simulink model "Robot"  (R2018a)
settings: Solver=VariableStepAuto  StartTime=0.0  StopTime=inf  FixedStep=1e-4  RelTol=1e-3  EnableMultiTasking=on
values from neighbouring files (symbols this model uses):
  CM730_acc_center = (4 * 9.80665)    (= 39.2266)    [CM730.m]
  CM730_acc_gain = 512 / CM730_acc_center    (= 13.0523675261)    [CM730.m]
  CM730_gyro_center = (1600 / 360 * 2 * pi)    (= 27.9252680319)    [CM730.m]
  CM730_gyro_gain = 512 / CM730_gyro_center    (= 18.3346494442)    [CM730.m]
  CM730_sample_time = 1e-3    (= 0.001)    [CM730.m]
  FSR_max = 254    [FSR.m]
  FSR_no_load = 255    [FSR.m]
  FSR_sample_time = 0.001    [FSR.m]
  FSR_scale = 1000    [FSR.m]
  g = 0    [Euler.m]
  MX106_Te = 1/1000    (= 0.001)    [MX106_init.m]
  MX28_inertia = 9e-8 * MX28_reduction^2    (= 0.0033385284)    [MX28_init.m]
  MX28_Te = 1/1000    (= 0.001)    [MX28_init.m]
  posZero_ID1 = posZero(1)    [Robot_init.m]
  posZero_ID10 = posZero(14)    [Robot_init.m]
  posZero_ID11 = posZero(9)    [Robot_init.m]
  posZero_ID12 = posZero(15)    [Robot_init.m]
  posZero_ID13 = posZero(10)    [Robot_init.m]
  posZero_ID14 = posZero(16)    [Robot_init.m]
  posZero_ID15 = posZero(11)    [Robot_init.m]
  posZero_ID16 = posZero(17)    [Robot_init.m]
  posZero_ID17 = posZero(12)    [Robot_init.m]
  posZero_ID18 = posZero(18)    [Robot_init.m]
  posZero_ID19 = posZero(19)    [Robot_init.m]
  posZero_ID2 = posZero(4)    [Robot_init.m]
  posZero_ID20 = posZero(20)    [Robot_init.m]
  posZero_ID3 = posZero(2)    [Robot_init.m]
  posZero_ID4 = posZero(5)    [Robot_init.m]
  posZero_ID5 = posZero(3)    [Robot_init.m]
  posZero_ID6 = posZero(6)    [Robot_init.m]
  posZero_ID7 = posZero(7)    [Robot_init.m]
  posZero_ID8 = posZero(13)    [Robot_init.m]
  posZero_ID9 = posZero(8)    [Robot_init.m]
  robot_chest_mass = 2385.0    (= 2385)    [Robot_init.m]
  robot_floor_friction_coeff = 0.6    [Robot_init.m]
  robot_floor_position_gain = -1e5    (= -100000)    [Robot_init.m]
  robot_floor_speed_gain = -1e3    (= -1000)    [Robot_init.m]
  robot_gravity = [0 0 0]    [Robot_init.m]
  robot_head_mass = 177.69    [Robot_init.m]
  robot_hip1_mass = 49.00    (= 49)    [Robot_init.m]
  robot_left_ankle_mass = 360.00    (= 360)    [Robot_init.m]
  robot_left_foot_mass = 267.00    (= 267)    [Robot_init.m]
  robot_left_forearm_mass = 248.00    (= 248)    [Robot_init.m]
  robot_left_hip2_mass = 358.00    (= 358)    [Robot_init.m]
  robot_left_lower_leg_mass = 129.00    (= 129)    [Robot_init.m]
  robot_left_shoulder_mass = 39.00    (= 39)    [Robot_init.m]
  robot_left_thigh_mass = 1263.00    (= 1263)    [Robot_init.m]
  robot_left_upper_arm_mass = 247.00    (= 247)    [Robot_init.m]
  robot_neck_mass = 90    [Robot_init.m]
  robot_right_ankle_mass = 360.00    (= 360)    [Robot_init.m]
  robot_right_foot_mass = 267.00    (= 267)    [Robot_init.m]
  robot_right_forearm_mass = 248.00    (= 248)    [Robot_init.m]
  robot_right_hip2_mass = 358.00    (= 358)    [Robot_init.m]
  robot_right_lower_leg_mass = 129.00    (= 129)    [Robot_init.m]
  robot_right_shoulder_mass = 39.00    (= 39)    [Robot_init.m]
  robot_right_thigh_mass = 263.00    (= 263)    [Robot_init.m]
  robot_right_upper_arm_mass = 247.00    (= 247)    [Robot_init.m]
  X = get(hObject,'Value')    [gui_kine.m]
  Y = get(hObject,'Value')    [gui_kine.m]
  Z = get(hObject,'Value')    [gui_kine.m]
libraries: sm_lib x167, fl_lib x128, nesl_utility x77, dspindex x1
(part 1 of 7)
settings Model: Creator=florent  LastModifiedBy=MRL
settings DataIOCC: SaveFormat=Array  SaveOutput=off  SignalLogging=off  DSMLogging=off  VisualizeSimOutput=off  SaveTime=off  OutputTimes=0:0.04:10
settings OptimizationCC: OptimizeBlockIOStorage=off  BufferReuse=off  GlobalBufferReuse=off  ExpressionFolding=off  LocalBlockOutputs=off  LifeSpan=inf  OptimizeDataStoreBuffers=off  BusAssignmentInplaceUpdate=off
settings DebuggingCC: SolverPrmCheckMsg=warning  StateNameClashWarn=warning  SFUnexpectedBacktrackingDiag=warning  SFNoUnconditionalDefaultTransitionDiag=warning  SFExecutionAtInitializationDiag=none
settings HardwareCC: ProdBitPerPointer=32  ProdBitPerSizeT=32  ProdBitPerPtrDiffT=32  ProdLargestAtomicFloat=None  ProdIntDivRoundTo=Undefined  ProdEndianess=Unspecified  ProdWordSize=32  ProdHWDeviceType=32-bit Generic
settings ModelReferenceCC: PropagateSignalLabelsOutOfModel=off
settings CodeAppCC: StateflowObjectComments=on
settings GRTTargetCC: TargetLangStandard=C89/C90 (ANSI)  GeneratePreprocessorConditionals=Disable all
settings ConfigComp: CovMetricSettings=dw  CovHtmlReporting=on  CovSaveCumulativeToWorkspaceVar=on  CovSaveSingleToWorkspaceVar=on  CovExternalEMLEnable=off  CovSFcnEnable=off
settings SimscapeCC: SimscapeNormalizeSystem=off
settings ConfigurationSet: Description=SimMechanics 2G
settings DiagnosticsConfigSet: SimMechanicsConflictingReferenceFrames=none

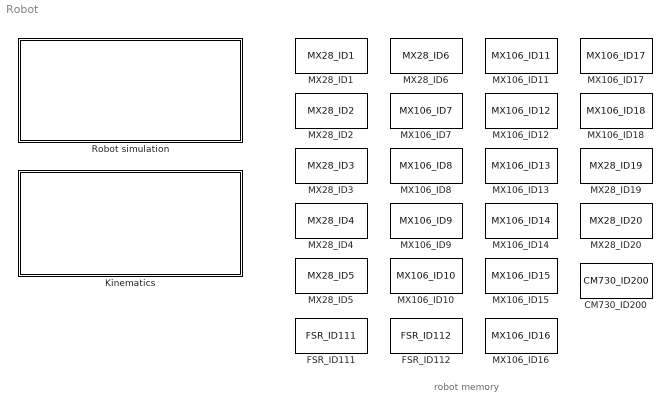
== system Robot ==
  note: robot memory
  CM730_ID200 : DataStoreMemory  DataStoreName=CM730_ID200  WriteAfterWriteMsg=error  InitialValue=CM730_default  VectorParams1D=off  ShowAdditionalParam=off  OutDataTypeStr=Bus: CM730_bus
  FSR_ID111 : DataStoreMemory  DataStoreName=FSR_ID111  WriteAfterWriteMsg=error  InitialValue=FSR_default  VectorParams1D=off  ShowAdditionalParam=off  OutDataTypeStr=Bus: FSR_bus
  FSR_ID112 : DataStoreMemory  DataStoreName=FSR_ID112  WriteAfterWriteMsg=error  InitialValue=FSR_default  VectorParams1D=off  ShowAdditionalParam=off  OutDataTypeStr=Bus: FSR_bus
  Kinematics : Subsystem
  MX106_ID10 : DataStoreMemory  DataStoreName=MX106_ID10  WriteAfterWriteMsg=error  InitialValue=MX106_default  VectorParams1D=off  ShowAdditionalParam=off  OutDataTypeStr=Bus: MX106_bus
  MX106_ID11 : DataStoreMemory  DataStoreName=MX106_ID11  WriteAfterWriteMsg=error  InitialValue=MX106_default  VectorParams1D=off  ShowAdditionalParam=off  OutDataTypeStr=Bus: MX106_bus
  MX106_ID12 : DataStoreMemory  DataStoreName=MX106_ID12  WriteAfterWriteMsg=error  InitialValue=MX106_default  VectorParams1D=off  ShowAdditionalParam=off  OutDataTypeStr=Bus: MX106_bus
  MX106_ID13 : DataStoreMemory  DataStoreName=MX106_ID13  WriteAfterWriteMsg=error  InitialValue=MX106_default  VectorParams1D=off  ShowAdditionalParam=off  OutDataTypeStr=Bus: MX106_bus
  MX106_ID14 : DataStoreMemory  DataStoreName=MX106_ID14  WriteAfterWriteMsg=error  InitialValue=MX106_default  VectorParams1D=off  ShowAdditionalParam=off  OutDataTypeStr=Bus: MX106_bus
  MX106_ID15 : DataStoreMemory  DataStoreName=MX106_ID15  WriteAfterWriteMsg=error  InitialValue=MX106_default  VectorParams1D=off  ShowAdditionalParam=off  OutDataTypeStr=Bus: MX106_bus
  MX106_ID16 : DataStoreMemory  DataStoreName=MX106_ID16  WriteAfterWriteMsg=error  InitialValue=MX106_default  VectorParams1D=off  ShowAdditionalParam=off  OutDataTypeStr=Bus: MX106_bus
  MX106_ID17 : DataStoreMemory  DataStoreName=MX106_ID17  WriteAfterWriteMsg=error  InitialValue=MX106_default  VectorParams1D=off  ShowAdditionalParam=off  OutDataTypeStr=Bus: MX106_bus
  MX106_ID18 : DataStoreMemory  DataStoreName=MX106_ID18  WriteAfterWriteMsg=error  InitialValue=MX106_default  VectorParams1D=off  ShowAdditionalParam=off  OutDataTypeStr=Bus: MX106_bus
  MX106_ID7 : DataStoreMemory  DataStoreName=MX106_ID7  WriteAfterWriteMsg=error  InitialValue=MX106_default  VectorParams1D=off  ShowAdditionalParam=off  OutDataTypeStr=Bus: MX106_bus
  MX106_ID8 : DataStoreMemory  DataStoreName=MX106_ID8  WriteAfterWriteMsg=error  InitialValue=MX106_default  VectorParams1D=off  ShowAdditionalParam=off  OutDataTypeStr=Bus: MX106_bus
  MX106_ID9 : DataStoreMemory  DataStoreName=MX106_ID9  WriteAfterWriteMsg=error  InitialValue=MX106_default  VectorParams1D=off  ShowAdditionalParam=off  OutDataTypeStr=Bus: MX106_bus
  MX28_ID1 : DataStoreMemory  DataStoreName=MX28_ID1  WriteAfterWriteMsg=error  InitialValue=MX28_default  VectorParams1D=off  ShowAdditionalParam=off  OutDataTypeStr=Bus: MX28_bus
  MX28_ID19 : DataStoreMemory  DataStoreName=MX28_ID19  WriteAfterWriteMsg=error  InitialValue=MX28_default  VectorParams1D=off  ShowAdditionalParam=off  OutDataTypeStr=Bus: MX28_bus
  MX28_ID2 : DataStoreMemory  DataStoreName=MX28_ID2  WriteAfterWriteMsg=error  InitialValue=MX28_default  VectorParams1D=off  ShowAdditionalParam=off  OutDataTypeStr=Bus: MX28_bus
  MX28_ID20 : DataStoreMemory  DataStoreName=MX28_ID20  WriteAfterWriteMsg=error  InitialValue=MX28_default  VectorParams1D=off  ShowAdditionalParam=off  OutDataTypeStr=Bus: MX28_bus
  MX28_ID3 : DataStoreMemory  DataStoreName=MX28_ID3  WriteAfterWriteMsg=error  InitialValue=MX28_default  VectorParams1D=off  ShowAdditionalParam=off  OutDataTypeStr=Bus: MX28_bus
  MX28_ID4 : DataStoreMemory  DataStoreName=MX28_ID4  WriteAfterWriteMsg=error  InitialValue=MX28_default  VectorParams1D=off  ShowAdditionalParam=off  OutDataTypeStr=Bus: MX28_bus
  MX28_ID5 : DataStoreMemory  DataStoreName=MX28_ID5  WriteAfterWriteMsg=error  InitialValue=MX28_default  VectorParams1D=off  ShowAdditionalParam=off  OutDataTypeStr=Bus: MX28_bus
  MX28_ID6 : DataStoreMemory  DataStoreName=MX28_ID6  WriteAfterWriteMsg=error  InitialValue=MX28_default  VectorParams1D=off  ShowAdditionalParam=off  OutDataTypeStr=Bus: MX28_bus
  Robot simulation : Subsystem

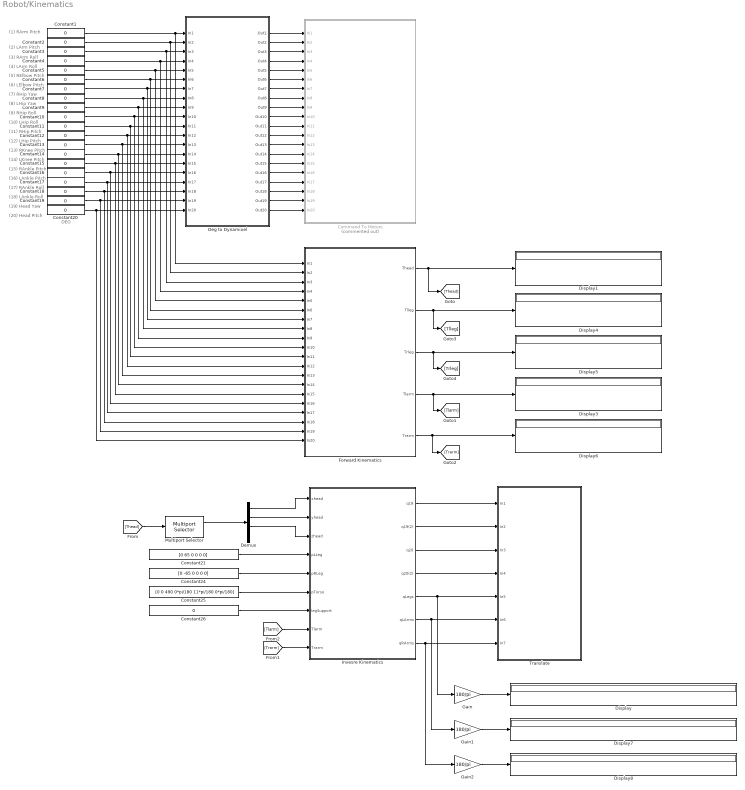
== system Robot/Kinematics ==
  note: (1) RArm Pitch
  note: (2) LArm Pitch
  note: (3) RArm Roll
  note: (4) LArm Roll
  note: (5) RElbow Pitch
  note: (6) LElbow Pitch
  note: (7) RHip Yaw
  note: (8) LHip Yaw
  note: (9) RHip Roll
  note: (10) LHip Roll
  note: (11) RHip Pitch
  note: (12) LHip Pitch
  note: (13) RKnee Pitch
  note: (14) LKnee Pitch
  note: (15) RAnkle Pitch
  note: (16) LAnkle Pitch
  note: (17) RAnkle Roll
  note: (18) LAnkle Roll
  note: (19) Head Yaw
  note: (20) Head Pitch
  note: DEG
  Command To Motors : Subsystem  Commented=on
  Constant{1..20} (20 alike) : Constant  Value=0  OutDataTypeStr=int16
  Constant21 : Constant  Value=[0 65 0 0 0 0]
  Constant24 : Constant  Value=[0 -65 0 0 0 0]
  Constant25 : Constant  Value="[0  0   490   0*pi/180   11*pi/180   0*pi/180]"
  Constant26 : Constant  Value=0
  Deg to Dynamixel : Subsystem
  Demux : Demux
  Display{,1,3..8} (8 alike) : Display
      Display1 settings: Format=bank
      Display3 settings: Format=bank
      Display4 settings: Format=bank
      Display5 settings: Format=bank
      Display6 settings: Format=bank
  Forward Kinematics : Subsystem
  Gain : Gain  Gain=180/pi
  Gain1 : Gain  Gain=180/pi
  Gain2 : Gain  Gain=180/pi
  Invesre Kinematics : Subsystem
  Multiport Selector : dspindex/Multiport Selector  rowsOrCols=Columns  idxCellArray={ 4,1}  idxErrMode=Clip Index
  Translate : Subsystem
  wires:
  Forward Kinematics/1(Thead) -> [Thead], Display1/1
  Forward Kinematics/2(Tlleg) -> Display4/1, [Tlleg]
  Forward Kinematics/3(Trleg) -> Display5/1, [Trleg]
  Constant1/1 -> Forward Kinematics/1(In1), Deg to Dynamixel/1(In1)
  Constant2/1 -> Forward Kinematics/2(In2), Deg to Dynamixel/2(In2)
  Constant3/1 -> Forward Kinematics/3(In3), Deg to Dynamixel/3(In3)
  Constant4/1 -> Forward Kinematics/4(In4), Deg to Dynamixel/4(In4)
  Constant5/1 -> Forward Kinematics/5(In5), Deg to Dynamixel/5(In5)
  Constant6/1 -> Forward Kinematics/6(In6), Deg to Dynamixel/6(In6)
  Constant7/1 -> Forward Kinematics/7(In7), Deg to Dynamixel/7(In7)
  Constant8/1 -> Forward Kinematics/8(In8), Deg to Dynamixel/8(In8)
  Constant9/1 -> Forward Kinematics/9(In9), Deg to Dynamixel/9(In9)
  Constant10/1 -> Forward Kinematics/10(In10), Deg to Dynamixel/10(In10)
  Constant11/1 -> Forward Kinematics/11(In11), Deg to Dynamixel/11(In11)
  Constant12/1 -> Forward Kinematics/12(In12), Deg to Dynamixel/12(In12)
  Constant13/1 -> Forward Kinematics/13(In13), Deg to Dynamixel/13(In13)
  Constant14/1 -> Forward Kinematics/14(In14), Deg to Dynamixel/14(In14)
  Constant15/1 -> Forward Kinematics/15(In15), Deg to Dynamixel/15(In15)
  Constant17/1 -> Forward Kinematics/17(In17), Deg to Dynamixel/17(In17)
  Constant18/1 -> Forward Kinematics/18(In18), Deg to Dynamixel/18(In18)
  Constant19/1 -> Forward Kinematics/19(In19), Deg to Dynamixel/19(In19)
  Deg to Dynamixel/1(Out1) -> Command To Motors/1(In1)
  Deg to Dynamixel/2(Out2) -> Command To Motors/2(In2)
  Deg to Dynamixel/3(Out3) -> Command To Motors/3(In3)
  Deg to Dynamixel/4(Out4) -> Command To Motors/4(In4)
  Deg to Dynamixel/5(Out5) -> Command To Motors/5(In5)
  Deg to Dynamixel/6(Out6) -> Command To Motors/6(In6)
  Deg to Dynamixel/7(Out7) -> Command To Motors/7(In7)
  Deg to Dynamixel/8(Out8) -> Command To Motors/8(In8)
  Deg to Dynamixel/9(Out9) -> Command To Motors/9(In9)
  Deg to Dynamixel/10(Out10) -> Command To Motors/10(In10)
  Deg to Dynamixel/11(Out11) -> Command To Motors/11(In11)
  Deg to Dynamixel/12(Out12) -> Command To Motors/12(In12)
  Deg to Dynamixel/13(Out13) -> Command To Motors/13(In13)
  Deg to Dynamixel/14(Out14) -> Command To Motors/14(In14)
  Deg to Dynamixel/15(Out15) -> Command To Motors/15(In15)
  Deg to Dynamixel/16(Out16) -> Command To Motors/16(In16)
  Deg to Dynamixel/17(Out17) -> Command To Motors/17(In17)
  Deg to Dynamixel/18(Out18) -> Command To Motors/18(In18)
  Deg to Dynamixel/19(Out19) -> Command To Motors/19(In19)
  Deg to Dynamixel/20(Out20) -> Command To Motors/20(In20)
  Constant16/1 -> Forward Kinematics/16(In16), Deg to Dynamixel/16(In16)
  [Thead] -> Multiport Selector/1
  Multiport Selector/1 -> Demux/1
  Demux/2 -> Invesre Kinematics/2(yhead)
  Demux/3 -> Invesre Kinematics/3(zhead)
  Invesre Kinematics/1(q19) -> Translate/1(In1)
  Invesre Kinematics/2(q19(2)) -> Translate/2(In2)
  Invesre Kinematics/3(q20) -> Translate/3(In3)
  Invesre Kinematics/4(q20(2)) -> Translate/4(In4)
  Demux/1 -> Invesre Kinematics/1(xhead)
  Constant20/1 -> Forward Kinematics/20(In20), Deg to Dynamixel/20(In20)
  Constant24/1 -> Invesre Kinematics/5(pRLeg)
  Constant25/1 -> Invesre Kinematics/6(pTorso)
  Constant26/1 -> Invesre Kinematics/7(legSupport)
  Invesre Kinematics/5(qLegs) -> Gain/1, Translate/5(In5)
  Gain/1 -> Display/1
  Constant21/1 -> Invesre Kinematics/4(pLLeg)
  Invesre Kinematics/6(qLArms) -> Gain1/1, Translate/6(In6)
  Invesre Kinematics/7(qRArms) -> Gain2/1, Translate/7(In7)
  Forward Kinematics/4(Tlarm) -> [Tlarm], Display3/1
  Forward Kinematics/5(Trarm) -> [Trarm], Display6/1
  Gain1/1 -> Display7/1
  Gain2/1 -> Display8/1
  [Trarm] -> Invesre Kinematics/9(Trarm)
  [Tlarm] -> Invesre Kinematics/8(Tlarm)

== system Robot/Robot simulation ==
  Chest : Subsystem
      mask init:
      | [ModelDir,~,~] = fileparts(which(gcs));
      | 
      | Block = [gcb '/Solid'];
      | STLFileName = [ModelDir filesep 'STL' filesep 'Chest.STL'];
      | if ~strcmp(get_param(Block,'ExtGeomFileName'),STLFileName)
      |     set_param(Block,'ExtGeomFileName',STLFileName);
      | end
  Free Fall Scope : Scope  Commented=on
  Free fall : sm_lib/Joints/6-DOF Joint  SenseConstraintForce=off  SenseConstraintForceX=off  SenseConstraintForceY=off  SenseConstraintForceZ=off  SenseConstraintTorque=off  SenseConstraintTorqueX=off  SenseConstraintTorqueY=off  SenseConstraintTorqueZ=off  SenseTotalForce=off  SenseTotalForceX=off  SenseTotalForceY=off  SenseTotalForceZ=off  SenseTotalTorque=off  SenseTotalTorqueX=off  SenseTotalTorqueY=off  SenseTotalTorqueZ=off  CompositeWrenchDir=FollowerOnBase  CompositeWrenchFrame=BaseFrame  PxEquilibriumPosition=0  PxEquilibriumPositionUnits=m  PxSpringStiffness=0  PxSpringStiffnessUnits=N/m  PxDampingCoefficient=0  PxDampingCoefficientUnits=N/(m/s)  PxTorqueActuationMode=NoTorque  PxMotionActuationMode=ComputedMotion  PxSensePosition=off  PxSenseVelocity=off  PxSenseAcceleration=off  PxSenseTorqueForce=off  PxPositionTargetSpecify=off  PxPositionTargetPriority=High  PxPositionTargetValue=0  PxPositionTargetValueUnits=m  PxVelocityTargetSpecify=off  PxVelocityTargetPriority=High  PxVelocityTargetValue=0  PxVelocityTargetValueUnits=m/s  PyEquilibriumPosition=0  PyEquilibriumPositionUnits=m  PySpringStiffness=0  PySpringStiffnessUnits=N/m  PyDampingCoefficient=0  PyDampingCoefficientUnits=N/(m/s)  PyTorqueActuationMode=NoTorque  PyMotionActuationMode=ComputedMotion  PySensePosition=off  PySenseVelocity=off  PySenseAcceleration=off  PySenseTorqueForce=off  PyPositionTargetSpecify=off  PyPositionTargetPriority=High  PyPositionTargetValue=0  PyPositionTargetValueUnits=m  PyVelocityTargetSpecify=off  PyVelocityTargetPriority=High  PyVelocityTargetValue=0  PyVelocityTargetValueUnits=m/s  PzEquilibriumPosition=0  PzEquilibriumPositionUnits=m  PzSpringStiffness=0  PzSpringStiffnessUnits=N/m  PzDampingCoefficient=0  PzDampingCoefficientUnits=N/(m/s)  PzTorqueActuationMode=NoTorque  PzMotionActuationMode=ComputedMotion  PzSensePosition=on  PzSenseVelocity=off  PzSenseAcceleration=off  PzSenseTorqueForce=off  PzPositionTargetSpecify=on  PzPositionTargetPriority=High  PzPositionTargetValue=512.5  PzPositionTargetValueUnits=mm  PzVelocityTargetSpecify=off  PzVelocityTargetPriority=High  PzVelocityTargetValue=0  PzVelocityTargetValueUnits=m/s  SphDefPosRotationMethod=None  SphDefPosRotationAngleUnits=deg  SphDefPosRotationStandardAxis=+Z  SphDefPosRotationAngle=0.0  SphDefPosRotationArbitraryAxis=[0 0 1]  SphDefPosFollAlignAxisA=+X  SphDefPosBaseAlignAxisA=+Y  SphDefPosFollAlignAxisB=+Y  SphDefPosBaseAlignAxisB=+Z  SphDefPosRotationSequenceAxes=FollowerAxes  SphDefPosRotationSequence=XYX  SphDefPosRotationSequenceAngles=[0 0 0]  SphDefPosRotationSequenceAnglesUnits=deg  SphDefPosRotationMatrix=[1 0 0; 0 1 0; 0 0 1]  SphEqPosRotationMethod=None  SphEqPosRotationAngleUnits=deg  SphEqPosRotationStandardAxis=+Z  SphEqPosRotationAngle=0.0  SphEqPosRotationArbitraryAxis=[0 0 1]  SphEqPosFollAlignAxisA=+X  SphEqPosBaseAlignAxisA=+Y  SphEqPosFollAlignAxisB=+Y  SphEqPosBaseAlignAxisB=+Z  SphEqPosRotationSequenceAxes=FollowerAxes  SphEqPosRotationSequence=XYX  SphEqPosRotationSequenceAngles=[0 0 0]  SphEqPosRotationSequenceAnglesUnits=deg  SphEqPosRotationMatrix=[1 0 0; 0 1 0; 0 0 1]  SphSpringStiffness=0  SphSpringStiffnessUnits=N*m/deg  SphDampingCoefficient=0  SphDampingCoefficientUnits=N*m/(deg/s)  SphActuateTorqueX=off  SphActuateTorqueY=off  SphActuateTorqueZ=off  SphActuateTorque=off  SphTorqueActuationMode=NoTorque  SphMotionActuationMode=ComputedMotion  SphActuationFrame=BaseFrame  SphSensePosition=off  SphSenseVelocityX=off  SphSenseVelocityY=off  SphSenseVelocityZ=off  SphSenseVelocity=off  SphSenseAccelerationX=off  SphSenseAccelerationY=off  SphSenseAccelerationZ=off  SphSenseAcceleration=off  SphSenseTorqueX=off  SphSenseTorqueY=off  SphSenseTorqueZ=off  SphSenseTorqueForce=off  SphSensingFrame=BaseFrame  SphPositionTargetRotationMethod=None  SphPositionTargetRotationAngleUnits=deg  SphPositionTargetRotationStandardAxis=+Z  SphPositionTargetRotationAngle=0.0  SphPositionTargetRotationArbitraryAxis=[0 0 1]  SphPositionTargetFollAlignAxisA=+X  SphPositionTargetBaseAlignAxisA=+Y  SphPositionTargetFollAlignAxisB=+Y  SphPositionTargetBaseAlignAxisB=+Z  SphPositionTargetRotationSequenceAxes=FollowerAxes  SphPositionTargetRotationSequence=XYX  SphPositionTargetRotationSequenceAngles=[0 0 0]  SphPositionTargetRotationSequenceAnglesUnits=deg  SphPositionTargetRotationMatrix=[1 0 0; 0 1 0; 0 0 1]  SphPositionTargetSpecify=off  SphPositionTargetPriority=High  SphVelocityTargetValue=[0 0 0]  SphVelocityTargetValueUnits=deg/s  SphVelocityTargetSpecify=off  SphVelocityTargetPriority=High  SphVelocityTargetInFollowerFrame=on
  Head : Subsystem
      mask init:
      | [ModelDir,~,~] = fileparts(which(gcs));
      | 
      | Block = [gcb '/Neck/Solid'];
      | STLFileName = [ModelDir filesep 'STL' filesep 'Neck.STL'];
      | if ~strcmp(get_param(Block,'ExtGeomFileName'),STLFileName)
      |     set_param(Block,'ExtGeomFileName',STLFileName);
      | end
      | 
      | Block = [gcb '/Head/Solid'];
      | STLFileName = [ModelDir filesep 'STL' filesep 'Head.STL'];
      | if ~strcmp(get_param(Block,'ExtGeomFileName'),STLFileName)
      |     set_param(Block,'ExtGeomFileName',STLFileName);
      | end
  Left Arm : Subsystem
      mask init:
      | [ModelDir,~,~] = fileparts(which(gcs));
      | 
      | Block = [gcb '/Left Shoulder/Solid'];
      | STLFileName = [ModelDir filesep 'STL' filesep 'Left_shoulder.STL'];
      | if ~strcmp(get_param(Block,'ExtGeomFileName'),STLFileName)
      |     set_param(Block,'ExtGeomFileName',STLFileName);
      | end
      | 
      | Block = [gcb '/Left Upper Arm/Solid'];
      | STLFileName = [ModelDir filesep 'STL' filesep 'Left_Arm.STL'];
      | if ~strcmp(get_param(Block,'ExtGeomFileName'),STLFileName)
      |     set_param(Block,'ExtGeomFileName',STLFileName);
      | end
      | 
      | Block = [gcb '/Left Forearm/Solid'];
      | STLFileName = [ModelDir filesep 'STL' filesep 'Left_Forearm.STL'];
      | if ~strcmp(get_param(Block,'ExtGeomFileName'),STLFileName)
      |     set_param(Block,'ExtGeomFileName',STLFileName);
      | end
  Left Leg : Subsystem
      mask init:
      | [ModelDir,~,~] = fileparts(which(gcs));
      | 
      | Block = [gcb '/Left Hip Yaw/Solid'];
      | STLFileName = [ModelDir filesep 'STL' filesep 'Hip1.STL'];
      | if ~strcmp(get_param(Block,'ExtGeomFileName'),STLFileName)
      |     set_param(Block,'ExtGeomFileName',STLFileName);
      | end
      | 
      | Block = [gcb '/Left Hip Roll/Solid'];
      | STLFileName = [ModelDir filesep 'STL' filesep 'Left_Hip2.STL'];
      | if ~strcmp(get_param(Block,'ExtGeomFileName'),STLFileName)
      |     set_param(Block,'ExtGeomFileName',STLFileName);
      | end
      | 
      | Block = [gcb '/Left Thigh/Solid'];
      | STLFileName = [ModelDir filesep 'STL' filesep 'Left_Thigh.STL'];
      | if ~strcmp(get_param(Block,'ExtGeomFileName'),STLFileName)
      |     set_param(Block,'ExtGeomFileName',STLFileName);
      | end
      | 
      | Block = [gcb '/Left Lower Leg/Solid'];
      | STLFileName = [ModelDir filesep 'STL' filesep 'Left_Lower_Leg.STL'];
      | if ~strcmp(get_param(Block,'ExtGeomFileName'),STLFileName)
      |     set_param(Block,'ExtGeomFileName',STLFileName);
      | end
      | 
      | Block = [gcb '/Left Ankle/Solid'];
      | STLFileName = [ModelDir filesep 'STL' filesep 'Left_Ankle.STL'];
      | if ~strcmp(get_param(Block,'ExtGeomFileName'),STLFileName)
      |     set_param(Block,'ExtGeomFileName',STLFileName);
      | end
      | 
      | Block = [gcb '/Left Foot/Solid'];
      | STLFileName = [ModelDir filesep 'STL' filesep 'Left_Foot.STL'];
      | if ~strcmp(get_param(Block,'ExtGeomFileName'),STLFileName)
      |     set_param(Block,'ExtGeomFileName',STLFileName);
      | end
  Mechanism Configuration : sm_lib/Utilities/Mechanism Configuration  UniformGravity=Constant  GravityVector=robot_gravity  GravityUnits=m/s^2  LinearizationDelta=0.001
  PS-Simulink Converter : nesl_utility/PS-Simulink Converter  Commented=on  PhysicalDomain=network_engine_domain  SubClassName=ps_output  LeftPortType=input  RightPortType=output  PseudoPeriodic=off  Frequencies=[]  Unit=m  AffineConversion=off
  Right Arm : Subsystem
      mask init:
      | [ModelDir,~,~] = fileparts(which(gcs));
      | 
      | Block = [gcb '/Right Shoulder/Solid'];
      | STLFileName = [ModelDir filesep 'STL' filesep 'Right_shoulder.STL'];
      | if ~strcmp(get_param(Block,'ExtGeomFileName'),STLFileName)
      |     set_param(Block,'ExtGeomFileName',STLFileName);
      | end
      | 
      | Block = [gcb '/Right Upper Arm/Solid'];
      | STLFileName = [ModelDir filesep 'STL' filesep 'Right_Arm.STL'];
      | if ~strcmp(get_param(Block,'ExtGeomFileName'),STLFileName)
      |     set_param(Block,'ExtGeomFileName',STLFileName);
      | end
      | 
      | Block = [gcb '/Right Forearm/Solid'];
      | STLFileName = [ModelDir filesep 'STL' filesep 'Right_Forearm.STL'];
      | if ~strcmp(get_param(Block,'ExtGeomFileName'),STLFileName)
      |     set_param(Block,'ExtGeomFileName',STLFileName);
      | end
  Right Leg : Subsystem
      mask init:
      | [ModelDir,~,~] = fileparts(which(gcs));
      | 
      | Block = [gcb '/Right Hip Yaw/Solid'];
      | STLFileName = [ModelDir filesep 'STL' filesep 'Hip1.STL'];
      | if ~strcmp(get_param(Block,'ExtGeomFileName'),STLFileName)
      |     set_param(Block,'ExtGeomFileName',STLFileName);
      | end
      | 
      | Block = [gcb '/Right Hip Roll/Solid'];
      | STLFileName = [ModelDir filesep 'STL' filesep 'Right_Hip2.STL'];
      | if ~strcmp(get_param(Block,'ExtGeomFileName'),STLFileName)
      |     set_param(Block,'ExtGeomFileName',STLFileName);
      | end
      | 
      | Block = [gcb '/Right Thigh/Solid'];
      | STLFileName = [ModelDir filesep 'STL' filesep 'Right_Thigh.STL'];
      | if ~strcmp(get_param(Block,'ExtGeomFileName'),STLFileName)
      |     set_param(Block,'ExtGeomFileName',STLFileName);
      | end
      | 
      | Block = [gcb '/Right Lower Leg/Solid'];
      | STLFileName = [ModelDir filesep 'STL' filesep 'Right_Lower_Leg.STL'];
      | if ~strcmp(get_param(Block,'ExtGeomFileName'),STLFileName)
      |     set_param(Block,'ExtGeomFileName',STLFileName);
      | end
      | 
      | Block = [gcb '/Right Ankle/Solid'];
      | STLFileName = [ModelDir filesep 'STL' filesep 'Right_Ankle.STL'];
      | if ~strcmp(get_param(Block,'ExtGeomFileName'),STLFileName)
      |     set_param(Block,'ExtGeomFileName',STLFileName);
      | end
      | 
      | Block = [gcb '/Right Foot/Solid'];
      | STLFileName = [ModelDir filesep 'STL' filesep 'Right_Foot.STL'];
      | if ~strcmp(get_param(Block,'ExtGeomFileName'),STLFileName)
      |     set_param(Block,'ExtGeomFileName',STLFileName);
      | end
  Rigid Transform : sm_lib/Frames and Transforms/Rigid Transform  Commented=on  TranslationMethod=Cartesian  TranslationStandardOffset=0  TranslationLengthUnit=mm  TranslationStandardAxis=+Z  TranslationCartesianOffset=[0 0 512]  TranslationROffset=0  TranslationROffsetUnits=m  TranslationZOffset=0  TranslationZOffsetUnits=m  TranslationThetaOffset=0  TranslationThetaOffsetUnits=deg  RotationMethod=None  RotationAngleUnits=deg  RotationStandardAxis=+Z  RotationAngle=0.0  RotationArbitraryAxis=[0 0 1]  FollAlignAxisA=+X  BaseAlignAxisA=+Y  FollAlignAxisB=+Y  BaseAlignAxisB=+Z  RotationSequenceAxes=FollowerAxes  RotationSequence=XYX  RotationSequenceAngles=[0 0 0]  RotationSequenceAnglesUnits=deg  RotationMatrix=[1 0 0; 0 1 0; 0 0 1]
  Robot Origin : sm_lib/Frames and Transforms/World Frame
  Solver Configuration : nesl_utility/Solver Configuration  PhysicalDomain=network_engine_domain  SubClassName=solver  LeftPortType=input  RightPortType=generic  Tones=[]  Harmonics=[]  SimulateNoise=off  Profile=off  UseLocalSampling=off  EnableSwitchedLinearOptims=on  FrequencyDomain=off  UseCCode=off  RelTol=0.001  AbsTol=1e-06  MinStep=1e-09  ToWorkspace=off  RevertToSquareIcSolve=off  NumHomotopyIterations=100  PhasorMode=off  PhasorModeNumHarmonics=1  DoDC=off  ResidualTolerance=1e-05  UseLocalSolver=off  LocalSolverChoice=NE_BACKWARD_EULER_ADVANCER  LocalSolverSampleTime=0.0001  DoFixedCost=off  MaxNonlinIter=3  MaxModeIter=2  LinearAlgebra=Sparse  EquationFormulation=NE_TIME_EF  DelaysMemoryBudget=1024  AutomaticFiltering=on  FilteringTimeConstant=0.001
  wires:
  PS-Simulink Converter/1 -> Free Fall Scope/1
  connections:
  Robot Origin/RConn1 -- Left Leg/LConn1 -- Solver Configuration/RConn1 -- Mechanism Configuration/RConn1 -- Right Leg/RConn1 -- Free fall/LConn1 -- Rigid Transform/LConn1
  Rigid Transform/RConn1 -- Free fall/RConn1 -- Chest/LConn3
  Head/LConn1 -- Chest/RConn1
  Chest/RConn2 -- Right Arm/LConn1
  Left Arm/RConn1 -- Chest/LConn1
  Right Leg/LConn1 -- Chest/RConn3
  Left Leg/RConn1 -- Chest/LConn2
  PS-Simulink Converter/LConn1 -- Free fall/RConn2

== system Robot/Kinematics/Command To Motors ==
  In1 : Inport
  In2 : Inport  Port=2
  In3 : Inport  Port=3
  In4 : Inport  Port=4
  In5 : Inport  Port=5
  In6 : Inport  Port=6
  In7 : Inport  Port=7
  In8 : Inport  Port=8
  In9 : Inport  Port=9
  In10 : Inport  Port=10
  In11 : Inport  Port=11
  In12 : Inport  Port=12
  In13 : Inport  Port=13
  In14 : Inport  Port=14
  In15 : Inport  Port=15
  In16 : Inport  Port=16
  In17 : Inport  Port=17
  In18 : Inport  Port=18
  In19 : Inport  Port=19
  In20 : Inport  Port=20
  Commands to Motors : Subsystem
  Mux : Mux  Inputs=20.
  Mux1 : Mux  Inputs=20.
  Read Position of Motors : Subsystem
  wires:
  Read Position of Motors/16(Out16) -> Mux/16
  Read Position of Motors/17(Out17) -> Mux/17
  In19/1 -> Mux1/19, Commands to Motors/19(In19)
  Read Position of Motors/9(Out9) -> Mux/9
  Read Position of Motors/5(Out5) -> Mux/5
  Read Position of Motors/6(Out6) -> Mux/6
  Read Position of Motors/1(Out1) -> Mux/1
  Read Position of Motors/8(Out8) -> Mux/8
  Read Position of Motors/7(Out7) -> Mux/7
  Read Position of Motors/15(Out15) -> Mux/15
  Read Position of Motors/14(Out14) -> Mux/14
  Read Position of Motors/3(Out3) -> Mux/3
  In18/1 -> Mux1/18, Commands to Motors/18(In18)
  Read Position of Motors/11(Out11) -> Mux/11
  Read Position of Motors/12(Out12) -> Mux/12
  Read Position of Motors/18(Out18) -> Mux/18
  Read Position of Motors/19(Out19) -> Mux/19
  In15/1 -> Mux1/15, Commands to Motors/15(In15)
  In13/1 -> Mux1/13, Commands to Motors/13(In13)
  In11/1 -> Mux1/11, Commands to Motors/11(In11)
  Read Position of Motors/2(Out2) -> Mux/2
  Read Position of Motors/20(Out20) -> Mux/20
  In9/1 -> Commands to Motors/9(In9)
  In14/1 -> Mux1/14, Commands to Motors/14(In14)
  In16/1 -> Mux1/16, Commands to Motors/16(In16)
  Read Position of Motors/13(Out13) -> Mux/13
  In1/1 -> Mux1/1, Commands to Motors/1(In1)
  In6/1 -> Commands to Motors/6(In6)
  In17/1 -> Mux1/17, Commands to Motors/17(In17)
  In7/1 -> Mux1/7, Commands to Motors/7(In7)
  Read Position of Motors/4(Out4) -> Mux/4
  In2/1 -> Mux1/2, Commands to Motors/2(In2)
  In10/1 -> Mux1/10, Commands to Motors/10(In10)
  In4/1 -> Mux1/4, Commands to Motors/4(In4)
  In3/1 -> Mux1/3, Commands to Motors/3(In3)
  In5/1 -> Mux1/6, Mux1/5, Commands to Motors/5(In5)
  Read Position of Motors/10(Out10) -> Mux/10
  In20/1 -> Mux1/20, Commands to Motors/20(In20)
  In12/1 -> Mux1/12, Commands to Motors/12(In12)
  In8/1 -> Mux1/9, Mux1/8, Commands to Motors/8(In8)

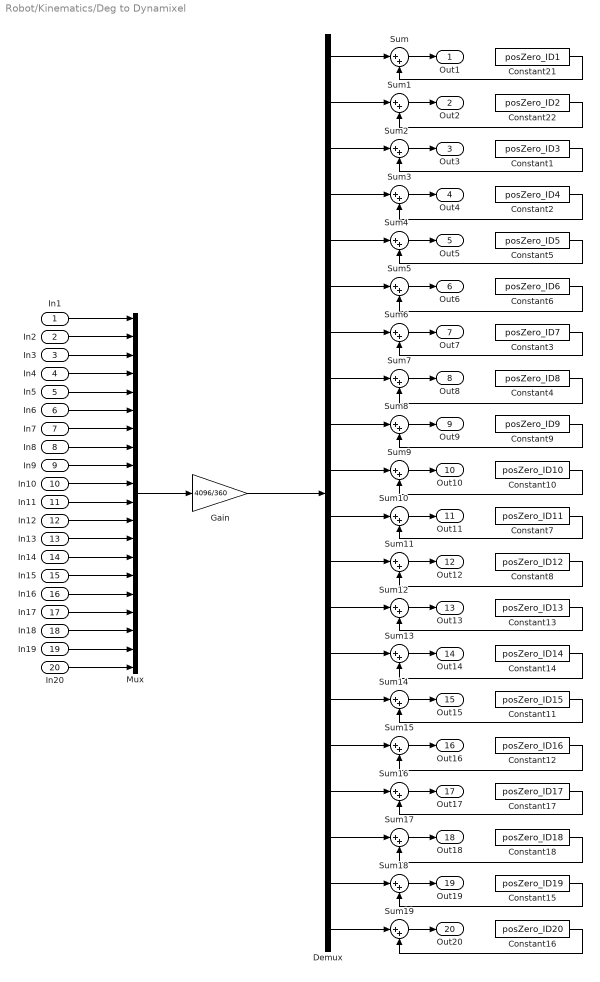
== system Robot/Kinematics/Deg to Dynamixel ==
  In1 : Inport
  In2 : Inport  Port=2
  In3 : Inport  Port=3
  In4 : Inport  Port=4
  In5 : Inport  Port=5
  In6 : Inport  Port=6
  In7 : Inport  Port=7
  In8 : Inport  Port=8
  In9 : Inport  Port=9
  In10 : Inport  Port=10
  In11 : Inport  Port=11
  In12 : Inport  Port=12
  In13 : Inport  Port=13
  In14 : Inport  Port=14
  In15 : Inport  Port=15
  In16 : Inport  Port=16
  In17 : Inport  Port=17
  In18 : Inport  Port=18
  In19 : Inport  Port=19
  In20 : Inport  Port=20
  Constant1 : Constant  Value=posZero_ID3  OutDataTypeStr=int16
  Constant10 : Constant  Value=posZero_ID10  OutDataTypeStr=int16
  Constant11 : Constant  Value=posZero_ID15  OutDataTypeStr=int16
  Constant12 : Constant  Value=posZero_ID16  OutDataTypeStr=int16
  Constant13 : Constant  Value=posZero_ID13  OutDataTypeStr=int16
  Constant14 : Constant  Value=posZero_ID14  OutDataTypeStr=int16
  Constant15 : Constant  Value=posZero_ID19  OutDataTypeStr=int16
  Constant16 : Constant  Value=posZero_ID20  OutDataTypeStr=int16
  Constant17 : Constant  Value=posZero_ID17  OutDataTypeStr=int16
  Constant18 : Constant  Value=posZero_ID18  OutDataTypeStr=int16
  Constant2 : Constant  Value=posZero_ID4  OutDataTypeStr=int16
  Constant21 : Constant  Value=posZero_ID1  OutDataTypeStr=int16
  Constant22 : Constant  Value=posZero_ID2  OutDataTypeStr=int16
  Constant3 : Constant  Value=posZero_ID7  OutDataTypeStr=int16
  Constant4 : Constant  Value=posZero_ID8  OutDataTypeStr=int16
  Constant5 : Constant  Value=posZero_ID5  OutDataTypeStr=int16
  Constant6 : Constant  Value=posZero_ID6  OutDataTypeStr=int16
  Constant7 : Constant  Value=posZero_ID11  OutDataTypeStr=int16
  Constant8 : Constant  Value=posZero_ID12  OutDataTypeStr=int16
  Constant9 : Constant  Value=posZero_ID9  OutDataTypeStr=int16
  Demux : Demux  Outputs=20
  Gain : Gain  Gain=4096/360  SaturateOnIntegerOverflow=on  OutDataTypeStr=Inherit: Same as input
  Mux : Mux  Inputs=20
  Sum{,1..19} (20 alike) : Sum  Inputs=|++
  Out1 : Outport
  Out2 : Outport  Port=2
  Out3 : Outport  Port=3
  Out4 : Outport  Port=4
  Out5 : Outport  Port=5
  Out6 : Outport  Port=6
  Out7 : Outport  Port=7
  Out8 : Outport  Port=8
  Out9 : Outport  Port=9
  Out10 : Outport  Port=10
  Out11 : Outport  Port=11
  Out12 : Outport  Port=12
  Out13 : Outport  Port=13
  Out14 : Outport  Port=14
  Out15 : Outport  Port=15
  Out16 : Outport  Port=16
  Out17 : Outport  Port=17
  Out18 : Outport  Port=18
  Out19 : Outport  Port=19
  Out20 : Outport  Port=20
  wires:
  In1/1 -> Mux/1
  In2/1 -> Mux/2
  In3/1 -> Mux/3
  In4/1 -> Mux/4
  In5/1 -> Mux/5
  In6/1 -> Mux/6
  In7/1 -> Mux/7
  In8/1 -> Mux/8
  In9/1 -> Mux/9
  In10/1 -> Mux/10
  In11/1 -> Mux/11
  In12/1 -> Mux/12
  In13/1 -> Mux/13
  In14/1 -> Mux/14
  In15/1 -> Mux/15
  In16/1 -> Mux/16
  In17/1 -> Mux/17
  In18/1 -> Mux/18
  In19/1 -> Mux/19
  In20/1 -> Mux/20
  Mux/1 -> Gain/1
  Gain/1 -> Demux/1
  Demux/1 -> Sum/1
  Constant21/1 -> Sum/2
  Sum/1 -> Out1/1
  Demux/2 -> Sum1/1
  Constant22/1 -> Sum1/2
  Sum1/1 -> Out2/1
  Sum3/1 -> Out4/1
  Constant2/1 -> Sum3/2
  Demux/4 -> Sum3/1
  Sum2/1 -> Out3/1
  Constant1/1 -> Sum2/2
  Demux/3 -> Sum2/1
  Demux/7 -> Sum6/1
  Constant3/1 -> Sum6/2
  Sum6/1 -> Out7/1
  Demux/8 -> Sum7/1
  Constant4/1 -> Sum7/2
  Sum7/1 -> Out8/1
  Sum5/1 -> Out6/1
  Constant6/1 -> Sum5/2
  Demux/6 -> Sum5/1
  Sum4/1 -> Out5/1
  Constant5/1 -> Sum4/2
  Demux/5 -> Sum4/1
  Demux/13 -> Sum12/1
  Constant13/1 -> Sum12/2
  Sum12/1 -> Out13/1
  Demux/14 -> Sum13/1
  Constant14/1 -> Sum13/2
  Sum13/1 -> Out14/1
  Sum15/1 -> Out16/1
  Constant12/1 -> Sum15/2
  Demux/16 -> Sum15/1
  Sum14/1 -> Out15/1
  Constant11/1 -> Sum14/2
  Demux/15 -> Sum14/1
  Demux/11 -> Sum10/1
  Constant7/1 -> Sum10/2
  Sum10/1 -> Out11/1
  Demux/12 -> Sum11/1
  Constant8/1 -> Sum11/2
  Sum11/1 -> Out12/1
  Sum9/1 -> Out10/1
  Constant10/1 -> Sum9/2
  Demux/10 -> Sum9/1
  Sum8/1 -> Out9/1
  Constant9/1 -> Sum8/2
  Demux/9 -> Sum8/1
  Demux/19 -> Sum18/1
  Constant15/1 -> Sum18/2
  Sum18/1 -> Out19/1
  Demux/20 -> Sum19/1
  Constant16/1 -> Sum19/2
  Sum19/1 -> Out20/1
  Sum17/1 -> Out18/1
  Constant18/1 -> Sum17/2
  Demux/18 -> Sum17/1
  Sum16/1 -> Out17/1
  Constant17/1 -> Sum16/2
  Demux/17 -> Sum16/1

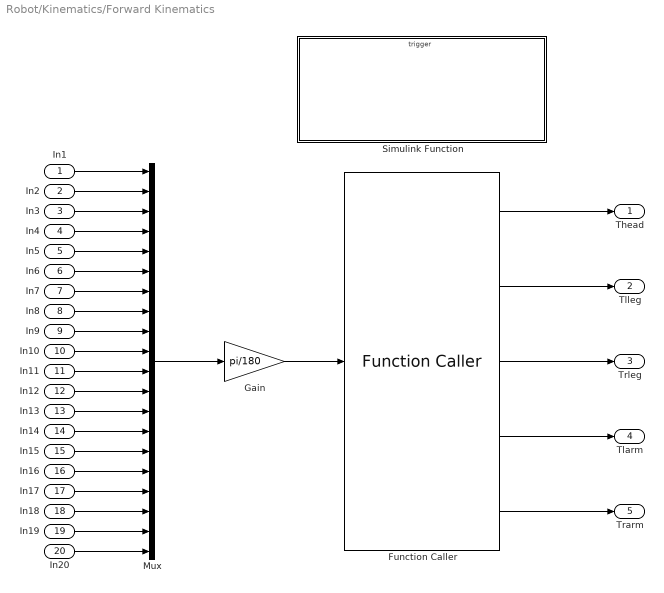
== system Robot/Kinematics/Forward Kinematics ==
  In1 : Inport
  In2 : Inport  Port=2
  In3 : Inport  Port=3
  In4 : Inport  Port=4
  In5 : Inport  Port=5
  In6 : Inport  Port=6
  In7 : Inport  Port=7
  In8 : Inport  Port=8
  In9 : Inport  Port=9
  In10 : Inport  Port=10
  In11 : Inport  Port=11
  In12 : Inport  Port=12
  In13 : Inport  Port=13
  In14 : Inport  Port=14
  In15 : Inport  Port=15
  In16 : Inport  Port=16
  In17 : Inport  Port=17
  In18 : Inport  Port=18
  In19 : Inport  Port=19
  In20 : Inport  Port=20
  Function Caller : FunctionCaller  FunctionPrototype=[Thead,Trleg,Tlleg,Trarm,Tlarm] = Transform(q)
  Gain : Gain  Gain=pi/180  OutDataTypeStr=double  SaturateOnIntegerOverflow=on
  Mux : Mux  Inputs=20
  Simulink Function : Subsystem  TreatAsAtomicUnit=on
  Thead : Outport
  Tlleg : Outport  Port=2
  Trleg : Outport  Port=3
  Tlarm : Outport  Port=4
  Trarm : Outport  Port=5
  wires:
  Gain/1 -> Function Caller/1
  Function Caller/1 -> Thead/1
  Function Caller/3 -> Trleg/1
  Function Caller/2 -> Tlleg/1
  In1/1 -> Mux/1
  In2/1 -> Mux/2
  In3/1 -> Mux/3
  In4/1 -> Mux/4
  In5/1 -> Mux/5
  In6/1 -> Mux/6
  In7/1 -> Mux/7
  In8/1 -> Mux/8
  In9/1 -> Mux/9
  In10/1 -> Mux/10
  In11/1 -> Mux/11
  In12/1 -> Mux/12
  In13/1 -> Mux/13
  In14/1 -> Mux/14
  In15/1 -> Mux/15
  In16/1 -> Mux/16
  In17/1 -> Mux/17
  In18/1 -> Mux/18
  In19/1 -> Mux/19
  In20/1 -> Mux/20
  Mux/1 -> Gain/1
  Function Caller/4 -> Tlarm/1
  Function Caller/5 -> Trarm/1

== system Robot/Kinematics/Invesre Kinematics ==
  xhead : Inport
  yhead : Inport  Port=2
  zhead : Inport  Port=3
  pLLeg : Inport  Port=4
  pRLeg : Inport  Port=5
  pTorso : Inport  Port=6
  legSupport : Inport  Port=7
  Tlarm : Inport  Port=8
  Trarm : Inport  Port=9
  Function Caller : FunctionCaller  FunctionPrototype=[q1,q2,q3,q4,qLegs,qLArms,qRArms] = InverseTransform(xhead,yhead,zhead,pLLeg,pRLeg,pTorso,legSupport,transLArm,transRArm)
  Simulink Function : Subsystem  TreatAsAtomicUnit=on
  q19 : Outport
  q19(2) : Outport  Port=2
  q20 : Outport  Port=3
  q20(2) : Outport  Port=4
  qLegs : Outport  Port=5
  qLArms : Outport  Port=6
  qRArms : Outport  Port=7
  wires:
  Function Caller/1 -> q19/1
  Function Caller/2 -> q19(2)/1
  Function Caller/3 -> q20/1
  xhead/1 -> Function Caller/1
  yhead/1 -> Function Caller/2
  zhead/1 -> Function Caller/3
  Function Caller/4 -> q20(2)/1
  Function Caller/5 -> qLegs/1
  pLLeg/1 -> Function Caller/4
  pRLeg/1 -> Function Caller/5
  pTorso/1 -> Function Caller/6
  legSupport/1 -> Function Caller/7
  Tlarm/1 -> Function Caller/8
  Trarm/1 -> Function Caller/9
  Function Caller/6 -> qLArms/1
  Function Caller/7 -> qRArms/1

== system Robot/Kinematics/Translate ==
  In1 : Inport
  In2 : Inport  Port=2
  In3 : Inport  Port=3
  In4 : Inport  Port=4
  In5 : Inport  Port=5
  In6 : Inport  Port=6
  In7 : Inport  Port=7
  Deg to Dynamixel : Subsystem
  Subsystem : Subsystem
  wires:
  In2/1 -> Deg to Dynamixel/2(In2)
  In4/1 -> Deg to Dynamixel/4(In4)
  In3/1 -> Deg to Dynamixel/3(In3)
  In1/1 -> Deg to Dynamixel/1(In1)
  In5/1 -> Deg to Dynamixel/5(In5)
  In6/1 -> Deg to Dynamixel/6(In6)
  In7/1 -> Deg to Dynamixel/7(In7)
  Deg to Dynamixel/1(Out1) -> Subsystem/1(In1)
  Deg to Dynamixel/2(Out2) -> Subsystem/2(In2)
  Deg to Dynamixel/3(Out3) -> Subsystem/3(In3)
  Deg to Dynamixel/4(Out4) -> Subsystem/4(In4)
  Deg to Dynamixel/5(Out5) -> Subsystem/5(In5)
  Deg to Dynamixel/6(Out6) -> Subsystem/6(In6)
  Deg to Dynamixel/7(Out7) -> Subsystem/7(In7)
  Deg to Dynamixel/8(Out8) -> Subsystem/8(In8)
  Deg to Dynamixel/9(Out9) -> Subsystem/9(In9)
  Deg to Dynamixel/10(Out10) -> Subsystem/10(In10)
  Deg to Dynamixel/11(Out11) -> Subsystem/11(In11)
  Deg to Dynamixel/12(Out12) -> Subsystem/12(In12)
  Deg to Dynamixel/13(Out13) -> Subsystem/13(In13)
  Deg to Dynamixel/14(Out14) -> Subsystem/14(In14)
  Deg to Dynamixel/15(Out15) -> Subsystem/15(In15)
  Deg to Dynamixel/16(Out16) -> Subsystem/16(In16)
  Deg to Dynamixel/17(Out17) -> Subsystem/17(In17)
  Deg to Dynamixel/18(Out18) -> Subsystem/18(In18)
  Deg to Dynamixel/19(Out19) -> Subsystem/19(In19)
  Deg to Dynamixel/20(Out20) -> Subsystem/20(In20)
  Deg to Dynamixel/21(Out21) -> Subsystem/21(In21)
  Deg to Dynamixel/22(Out22) -> Subsystem/22(In22)
  Deg to Dynamixel/23(Out23) -> Subsystem/23(In23)
  Deg to Dynamixel/24(Out24) -> Subsystem/24(In24)
  Deg to Dynamixel/25(Out25) -> Subsystem/25(In25)
  Deg to Dynamixel/26(Out26) -> Subsystem/26(In26)
